simulink model "VerificationSwitch"  (R2018a)
settings: Solver=ode4  StartTime=0.0  StopTime=Tfinal  FixedStep=Ts  RelTol=1e-3  EnableMultiTasking=on
values from neighbouring files (symbols this model uses):
  delta = 0    [sim_parameters.m]
  ma1 = 0.9    [sim_parameters.m]
  phase = 0    [sim_parameters.m]
  Ts = 1e-7    (= 1e-07)    [sim_parameters.m]
  wout = 2*pi*fout    (= 314.159265359)    [sim_parameters.m]
libraries: powerlib_meascontrol x1, powerlib x1
settings Model: SimulationMode=accelerator  Creator=ugurm  LastModifiedBy=enes_
settings DataIOCC: LimitDataPoints=on  SaveFormat=Array
settings OptimizationCC: EfficientMapNaN2IntZero=off  LifeSpan=inf
settings DebuggingCC: UnderspecifiedInitializationDetection=Classic  MergeDetectMultiDrivingBlocksExec=none  SolverPrmCheckMsg=warning  StateNameClashWarn=warning  SFUnexpectedBacktrackingDiag=warning  SFNoUnconditionalDefaultTransitionDiag=warning  SFExecutionAtInitializationDiag=none
settings HardwareCC: ProdBitPerPointer=32  ProdBitPerSizeT=32  ProdBitPerPtrDiffT=32  ProdLargestAtomicFloat=None  ProdIntDivRoundTo=Undefined  ProdEndianess=Unspecified  ProdWordSize=32  ProdHWDeviceType=32-bit Generic  TargetBitPerPointer=64  TargetBitPerSizeT=64  TargetBitPerPtrDiffT=64  TargetLongLongMode=on  TargetIntDivRoundTo=Zero  TargetEndianess=LittleEndian  TargetWordSize=64  TargetHWDeviceType=MATLAB Host  ProdEqTarget=off
settings ModelReferenceCC: PropagateSignalLabelsOutOfModel=off
settings CodeAppCC: MaxIdLength=128
settings GRTTargetCC: TargetLangStandard=C89/C90 (ANSI)  CombineOutputUpdateFcns=off  GRTInterface=on
settings ConfigComp: CovMetricSettings=dw  CovHtmlReporting=on  CovSaveCumulativeToWorkspaceVar=on  CovSaveSingleToWorkspaceVar=on  CovExternalEMLEnable=off
settings SimscapeCC: SimscapeNormalizeSystem=off

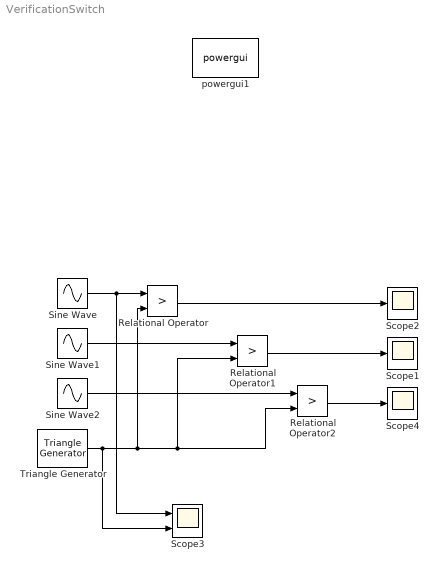
== system VerificationSwitch ==
  Relational Operator : RelationalOperator  Operator=>  OutDataTypeStr=boolean  RndMeth=Simplest
  Relational Operator1 : RelationalOperator  Operator=>  OutDataTypeStr=boolean  RndMeth=Simplest
  Relational Operator2 : RelationalOperator  Operator=>  OutDataTypeStr=boolean  RndMeth=Simplest
  Scope1 : Scope
  Scope2 : Scope
  Scope3 : Scope  NumInputPorts=2
  Scope4 : Scope
  Sine Wave : Sin  Amplitude=ma1  Frequency=wout  Phase=delta  SampleTime=0
  Sine Wave1 : Sin  Amplitude=ma1  Frequency=wout  Phase=-2*pi/3+delta  SampleTime=0
  Sine Wave2 : Sin  Amplitude=ma1  Frequency=wout  Phase=2*pi/3+delta  SampleTime=0
  Triangle Generator : powerlib_meascontrol/Pulse & Signal Generators/Triangle Generator  Freq=fsw  Phase=phase  Ts=Ts
  powergui1 : powerlib/powergui  Priority=1  SimulationMode=Discrete  SampleTime=Ts  frequency=60  Iterations=50  frequencyindice=0  Pbase=100e6  ErrMax=1e-4  UnitsV=kV  UnitsW=MW  buscounter=0  FunctionMessages=off  echomessages=off  EnableUseOfTLC=off  CurrentSourceSwitches=off  DisableSnubberDevices=off  DisableRonSwitches=off  DisableVfSwitches=off  DisplayEquations=off  SolverType=Tustin  Interpol=off  ExternalGateDelay=off  methode=off  Ts=0  x0status=blocks  SPID=off  SwTol=0  HookPort=off  RestoreLinks=warning  ResistiveCurrentMeasurement=off  Frange=[0:2:500]  Ylog=off  Xlog=on  ShowGrid=off  save=off  variable=ZData  structure=SA  ZoomFFT=off  StartTime=0  cycles=4  DisplayStyle=4  fundamental=50  FreqAxis=off  MaxFrequency=300000  frequencyindicesteady=1  RmsSteady=1  display=off
  wires:
  Sine Wave1/1 -> Relational Operator1/1
  Sine Wave/1 -> Relational Operator/1, Scope3/1
  Sine Wave2/1 -> Relational Operator2/1
  Triangle Generator/1 -> Scope3/2, Relational Operator/2, Relational Operator1/2, Relational Operator2/2
  Relational Operator/1 -> Scope2/1
  Relational Operator1/1 -> Scope1/1
  Relational Operator2/1 -> Scope4/1
